simulink model "transfer_function"  (R2018b)
settings: Solver=VariableStepAuto  StartTime=0.0  StopTime=10.0  RelTol=1e-3
libraries: cstblocks x1
settings Model: Creator=My NoteBook  LastModifiedBy=Tara

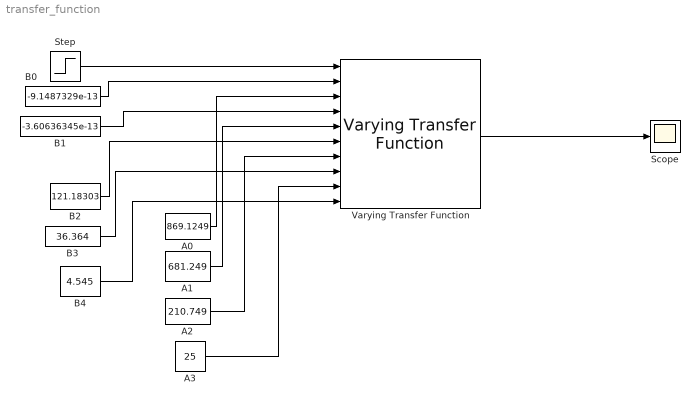
== system transfer_function ==
  "A0 " : Constant  Value=869.1249
  "A1 " : Constant  Value=681.249
  A2 : Constant  Value=210.749
  "A3 " : Constant  Value=25
  "B0 " : Constant  Value=-9.1487329e-13
  "B1 " : Constant  Value=-3.60636345e-13
  "B2 " : Constant  Value=121.18303
  B3 : Constant  Value=36.364
  "B4 " : Constant  Value=4.545
  Scope : Scope
  Step : Step  SampleTime=0
  Varying Transfer Function : cstblocks/Linear Parameter Varying/Varying Transfer Function  N=4
      settings: SourceProductName=Control System Toolbox
  wires:
  Step/1 -> Varying Transfer Function/1
  "B0 "/1 -> Varying Transfer Function/2
  "A0 "/1 -> Varying Transfer Function/3
  "B1 "/1 -> Varying Transfer Function/4
  "A1 "/1 -> Varying Transfer Function/5
  "B2 "/1 -> Varying Transfer Function/6
  B3/1 -> Varying Transfer Function/8
  A2/1 -> Varying Transfer Function/7
  "A3 "/1 -> Varying Transfer Function/9
  "B4 "/1 -> Varying Transfer Function/10
  Varying Transfer Function/1 -> Scope/1
